simulink model "adaptive"  (R2021b)
settings: Solver=VariableStepAuto  StartTime=0.0  StopTime=10.0  RelTol=1e-3
undefined symbols (not defined in the file): A, F, F_est, G, G_est, I, I_est, K, Kd, lambda
settings Model: Creator=simon  LastModifiedBy=buse
settings SolverCC: AlgebraicLoopSolver=TrustRegion
settings DebuggingCC: SFMachineParentedDataDiag=warning

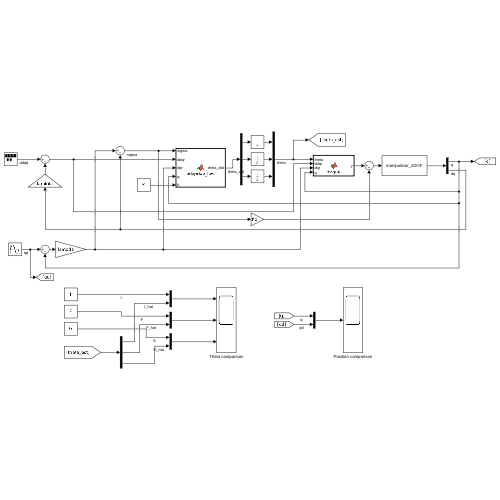
[thumbnail: Simulink's stored preview of the top-level diagram]
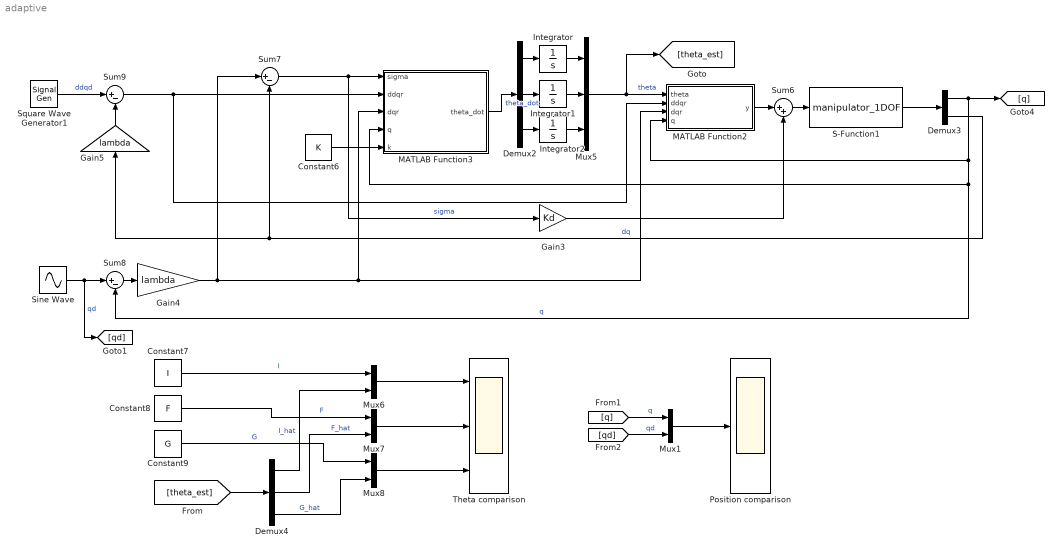
== system adaptive ==
  Constant6 : Constant  Value=K
  Constant7 : Constant  Value=I
  Constant8 : Constant  Value=F
  Constant9 : Constant  Value=G
  Demux2 : Demux  Outputs=3
  Demux3 : Demux  Outputs=2
  Demux4 : Demux  Outputs=3
  Gain3 : Gain  Gain=Kd
  Gain4 : Gain  Gain=lambda
  Gain5 : Gain  Gain=lambda
  Integrator : Integrator  InitialCondition=I_est
  Integrator1 : Integrator  InitialCondition=F_est
  Integrator2 : Integrator  InitialCondition=G_est
  MATLAB Function2 : MATLAB Function  TreatAsAtomicUnit=on
  MATLAB Function3 : MATLAB Function  TreatAsAtomicUnit=on
  Mux{1,6..8} (4 alike) : Mux  Inputs=2
  Mux5 : Mux  Inputs=3
  Position comparison : Scope
  S-Function1 : S-Function  FunctionName=manipulator_1DOF  Parameters=qi, dqi,I,F,G  SFunctionDeploymentMode=off  EnableBusSupport=off
  Sine Wave : Sin  Amplitude=A  Frequency=3.14  SampleTime=0
  Square Wave Generator1 : SignalGenerator  WaveForm=square  Amplitude=A  Units=rad/sec
  Sum6 : Sum  Inputs=|++
  Sum7 : Sum  Inputs=|+-
  Sum8 : Sum  Inputs=|+-
  Sum9 : Sum  Inputs=|+-
  Theta comparison : Scope  NumInputPorts=3
  wires:
  Demux2/2 -> Integrator1/1
  Demux2/1 -> Integrator/1
  Integrator1/1 -> Mux5/2
  Demux2/3 -> Integrator2/1
  Integrator2/1 -> Mux5/3
  Integrator/1 -> Mux5/1
  Mux5/1 -> [theta_est], MATLAB Function2/1(theta)  "theta"
  MATLAB Function3/1(theta_dot) -> Demux2/1  "theta_dot"
  MATLAB Function2/1(y) -> Sum6/1
  Sum6/1 -> S-Function1/1
  Gain3/1 -> Sum6/2
  Sum7/1 -> Gain3/1, MATLAB Function3/1(sigma)  "sigma"
  S-Function1/1 -> Demux3/1
  Demux3/1 -> [q], MATLAB Function2/4(q), Sum8/2, MATLAB Function3/4(q)  "q"
  Constant6/1 -> MATLAB Function3/5(k)
  Gain5/1 -> Sum9/2
  Demux3/2 -> Gain5/1, Sum7/2  "dq"
  Sum9/1 -> MATLAB Function2/2(ddqr), MATLAB Function3/2(ddqr)
  Square Wave Generator1/1 -> Sum9/1  "ddqd"
  Sine Wave/1 -> [qd], Sum8/1  "qd"
  Sum8/1 -> Gain4/1
  Gain4/1 -> Sum7/1, MATLAB Function2/3(dqr), MATLAB Function3/3(dqr)
  [theta_est] -> Demux4/1
  Mux6/1 -> Theta comparison/1
  Mux7/1 -> Theta comparison/2
  Mux8/1 -> Theta comparison/3
  Constant7/1 -> Mux6/1  "I"
  Constant8/1 -> Mux7/1  "F"
  Constant9/1 -> Mux8/1  "G"
  Demux4/1 -> Mux6/2  "I_hat"
  Demux4/2 -> Mux7/2  "F_hat"
  Demux4/3 -> Mux8/2  "G_hat"
  Mux1/1 -> Position comparison/1
  [q] -> Mux1/1  "q"
  [qd] -> Mux1/2  "qd"

== matlab function adaptive/MATLAB Function2 ==
  data: theta input; y output; ddqr input; dqr input; q input
function y = torque(theta, ddqr, dqr, q)
    y = [ddqr dqr sin(q)]*theta;

== matlab function adaptive/MATLAB Function3 ==
  data: sigma input; ddqr input; dqr input; q input; k input; theta_dot output size=3
function theta_dot = adaptive_law(sigma,ddqr,dqr,q,k)
    theta_dot = k*[ddqr;dqr;sin(q)];
